simulink model "FluidAndThermodynamics_simulink"  (R2022a)
settings: Solver=VariableStepAuto  StartTime=0.0  StopTime=10.0  RelTol=1e-3
settings Model: Creator=Anupp  LastModifiedBy=Anupp

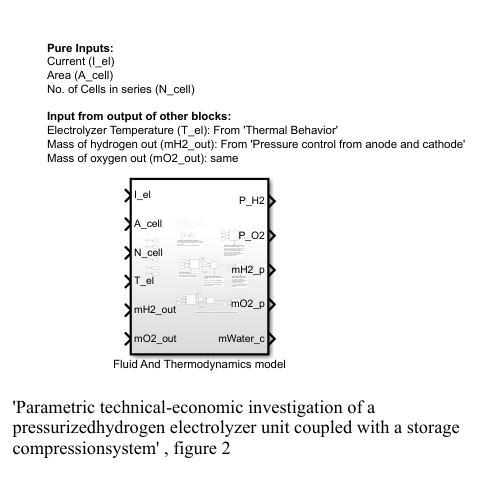
[thumbnail: Simulink's stored preview of the top-level diagram]
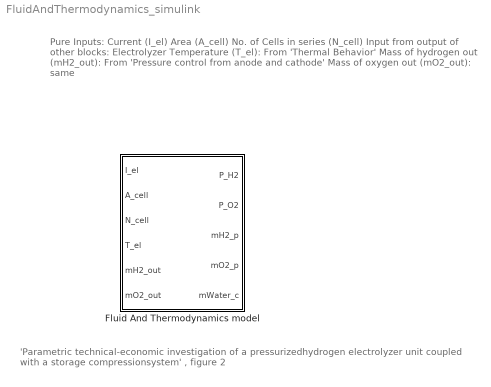
== system FluidAndThermodynamics_simulink ==
  note: Pure Inputs:
      | Current (I_el)
      | Area (A_cell)
      | No. of Cells in series (N_cell)
      |
      | Input from output of other blocks:
      | Electrolyzer Temperature (T_el): From 'Thermal Behavior'
      | Mass of hydrogen out (mH2_out): From 'Pressure control from anode and cathode'
      | Mass of oxygen out (mO2_out): same
  note: 'Parametric technical-economic investigation of a pressurizedhydrogen electrolyzer unit coupled with a storage compressionsystem' , figure 2
  Fluid And Thermodynamics model : Subsystem  TreatAsAtomicUnit=on

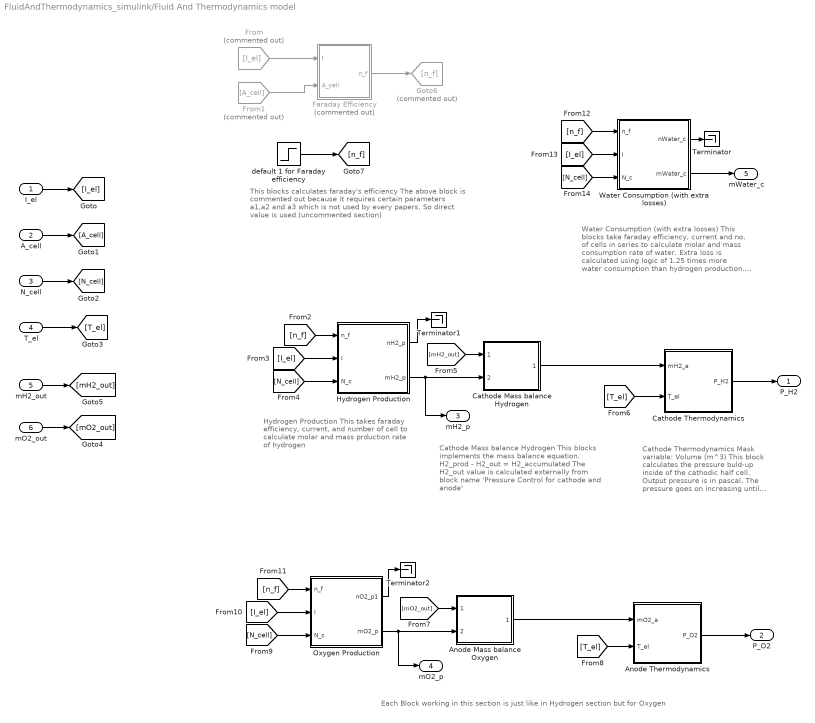
== system FluidAndThermodynamics_simulink/Fluid And Thermodynamics model ==
  note: Water Consumption (with extra losses)
      | This blocks take faraday efficiency, current and no. of cells in series to calculate molar and mass consumption rate of water.
      | Extra loss is calculated using logic of 1.25 times more water consumption than hydrogen production. Ideally, same moles of hydrgen production and water consumption takes place.
  note: This blocks calculates faraday's efficiency
      | The above block is commented out because it requires certain parameters a1,a2 and a3 which is not used by every papers.
      | So direct value is used (uncommented section)
  note: Each Block working in this section is just like in Hydrogen section but for Oxygen
  note: Cathode Thermodynamics
      | Mask variable: Volume (m^3)
      | This block calculates the pressure buld-up inside of the cathodic half cell. Output pressure is in pascal.
      | The pressure goes on increasing until the nominal pressure is reached.
  note: Cathode Mass balance Hydrogen
      | This blocks implements the mass balance equation.
      | H2_prod - H2_out = H2_accumulated
      |
      | The H2_out value is calculated externally from block name 'Pressure Control for cathode and anode'
  note: Hydrogen Production
      | This takes faraday efficiency, current, and number of cell to calculate molar and mass prduction rate of hydrogen
  I_el : Inport
  A_cell : Inport  Port=2
  N_cell : Inport  Port=3
  T_el : Inport  Port=4
  mH2_out : Inport  Port=5
  mO2_out : Inport  Port=6
  Anode Mass balance Oxygen : Subsystem
  Anode Thermodynamics : Subsystem  mask{V=0}
      mask prompts: V "Anode Volume"
  Cathode Mass balance Hydrogen : Subsystem
  Cathode Thermodynamics : Subsystem  mask{V=0}
      mask prompts: V "Cathode Volume"
  Faraday Efficiency : Subsystem  Commented=on  mask{a1=0, a2=0, a3=0}
      mask DialogControl DescTextVar Prompt: Define Faraday's efficiency parameters for alkaline electrolyser
  From : From  Commented=on  GotoTag=I_el
  From1 : From  Commented=on  GotoTag=A_cell
  Goto6 : Goto  Commented=on  GotoTag=n_f
  Hydrogen Production : Subsystem
  Oxygen Production : Subsystem
  Terminator : Terminator
  Terminator1 : Terminator
  Terminator2 : Terminator
  Water Consumption (with extra losses) : Subsystem
  default 1 for Faraday efficiency : Step  Time=0  SampleTime=0
  P_H2 : Outport
  P_O2 : Outport  Port=2
  mH2_p : Outport  Port=3
  mO2_p : Outport  Port=4
  mWater_c : Outport  Port=5
  wires:
  From1/1 -> Faraday Efficiency/2(A_cell)
  From/1 -> Faraday Efficiency/1(I)
  Cathode Mass balance Hydrogen/1(mH2_a) -> Cathode Thermodynamics/1(mH2_a)
  [n_f] -> Hydrogen Production/1(n_f)
  T_el/1 -> [T_el]
  [I_el] -> Water Consumption (with extra losses)/2(I)
  Hydrogen Production/2(mH2_p) -> mH2_p/1, Cathode Mass balance Hydrogen/2(mH2_p)
  N_cell/1 -> [N_cell]
  I_el/1 -> [I_el]
  [n_f] -> Oxygen Production/1(n_f)
  mO2_out/1 -> [mO2_out]
  Water Consumption (with extra losses)/2(mWater_c) -> mWater_c/1
  A_cell/1 -> [A_cell]
  mH2_out/1 -> [mH2_out]
  [I_el] -> Oxygen Production/2(I)
  [N_cell] -> Oxygen Production/3(N_c)
  [mH2_out] -> Cathode Mass balance Hydrogen/1(mH2_out)
  [N_cell] -> Hydrogen Production/3(N_c)
  Oxygen Production/2(mO2_p) -> mO2_p/1, Anode Mass balance Oxygen/2(mO2_p)
  [I_el] -> Hydrogen Production/2(I)
  Faraday Efficiency/1(n_f) -> Goto6/1
  [T_el] -> Cathode Thermodynamics/2(T_el)
  [N_cell] -> Water Consumption (with extra losses)/3(N_c)
  [n_f] -> Water Consumption (with extra losses)/1(n_f)
  [T_el] -> Anode Thermodynamics/2(T_el)
  Anode Mass balance Oxygen/1(mO2_a) -> Anode Thermodynamics/1(mO2_a)
  [mO2_out] -> Anode Mass balance Oxygen/1(mO2_out)
  Cathode Thermodynamics/1(P_H2) -> P_H2/1
  Anode Thermodynamics/1(P_O2) -> P_O2/1
  Water Consumption (with extra losses)/1(nWater_c) -> Terminator/1
  Hydrogen Production/1(nH2_p) -> Terminator1/1
  Oxygen Production/1(nO2_p1) -> Terminator2/1
  default 1 for Faraday efficiency/1 -> [n_f]

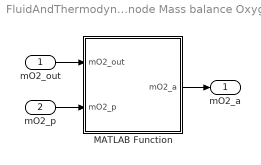
== system FluidAndThermodynamics_simulink/Fluid And Thermodynamics model/Anode Mass balance Oxygen ==
  mO2_out : Inport
  mO2_p : Inport  Port=2
  MATLAB Function : MATLAB Function  TreatAsAtomicUnit=on
  mO2_a : Outport
  wires:
  MATLAB Function/1(mO2_a) -> mO2_a/1
  mO2_p/1 -> MATLAB Function/2(mO2_p)
  mO2_out/1 -> MATLAB Function/1(mO2_out)

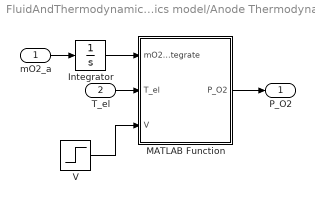
== system FluidAndThermodynamics_simulink/Fluid And Thermodynamics model/Anode Thermodynamics ==
  mO2_a : Inport
  T_el : Inport  Port=2
  Integrator : Integrator
  MATLAB Function : MATLAB Function  TreatAsAtomicUnit=on
  V : Step  Time=0  After=V  SampleTime=0
  P_O2 : Outport
  wires:
  T_el/1 -> MATLAB Function/2(T_el)
  mO2_a/1 -> Integrator/1
  Integrator/1 -> MATLAB Function/1(mO2_a_integrate)
  MATLAB Function/1(P_O2) -> P_O2/1
  V/1 -> MATLAB Function/3(V)

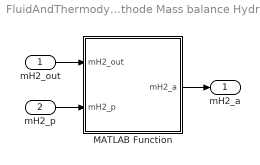
== system FluidAndThermodynamics_simulink/Fluid And Thermodynamics model/Cathode Mass balance Hydrogen ==
  mH2_out : Inport
  mH2_p : Inport  Port=2
  MATLAB Function : MATLAB Function  TreatAsAtomicUnit=on
  mH2_a : Outport
  wires:
  MATLAB Function/1(mH2_a) -> mH2_a/1
  mH2_p/1 -> MATLAB Function/2(mH2_p)
  mH2_out/1 -> MATLAB Function/1(mH2_out)

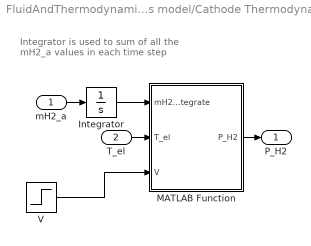
== system FluidAndThermodynamics_simulink/Fluid And Thermodynamics model/Cathode Thermodynamics ==
  note: Integrator is used to sum of all the mH2_a values in each time step
  mH2_a : Inport
  T_el : Inport  Port=2
  Integrator : Integrator
  MATLAB Function : MATLAB Function  TreatAsAtomicUnit=on
  V : Step  Time=0  After=V  SampleTime=0
  P_H2 : Outport
  wires:
  Integrator/1 -> MATLAB Function/1(mH2_a_integrate)
  MATLAB Function/1(P_H2) -> P_H2/1
  mH2_a/1 -> Integrator/1
  T_el/1 -> MATLAB Function/2(T_el)
  V/1 -> MATLAB Function/3(V)

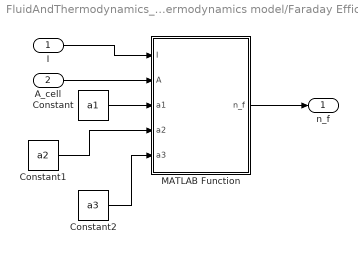
== system FluidAndThermodynamics_simulink/Fluid And Thermodynamics model/Faraday Efficiency ==
  I : Inport
  A_cell : Inport  Port=2
  Constant : Constant  Value=a1
  Constant1 : Constant  Value=a2
  Constant2 : Constant  Value=a3
  MATLAB Function : MATLAB Function  TreatAsAtomicUnit=on
  n_f : Outport
  wires:
  MATLAB Function/1(n_f) -> n_f/1
  Constant2/1 -> MATLAB Function/5(a3)
  Constant1/1 -> MATLAB Function/4(a2)
  A_cell/1 -> MATLAB Function/2(A)
  I/1 -> MATLAB Function/1(I)
  Constant/1 -> MATLAB Function/3(a1)

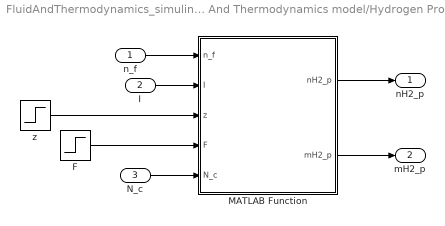
== system FluidAndThermodynamics_simulink/Fluid And Thermodynamics model/Hydrogen Production ==
  n_f : Inport
  I : Inport  Port=2
  N_c : Inport  Port=3
  F : Step  Time=0  After=96485  SampleTime=0
  MATLAB Function : MATLAB Function  TreatAsAtomicUnit=on
  z : Step  Time=0  After=2  SampleTime=0
  nH2_p : Outport
  mH2_p : Outport  Port=2
  wires:
  n_f/1 -> MATLAB Function/1(n_f)
  I/1 -> MATLAB Function/2(I)
  MATLAB Function/2(mH2_p) -> mH2_p/1
  N_c/1 -> MATLAB Function/5(N_c)
  F/1 -> MATLAB Function/4(F)
  z/1 -> MATLAB Function/3(z)
  MATLAB Function/1(nH2_p) -> nH2_p/1

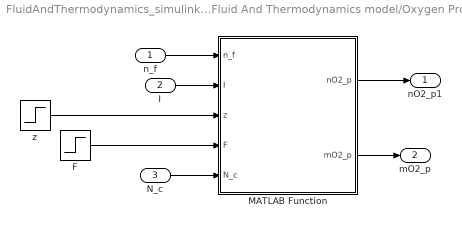
== system FluidAndThermodynamics_simulink/Fluid And Thermodynamics model/Oxygen Production ==
  n_f : Inport
  I : Inport  Port=2
  N_c : Inport  Port=3
  F : Step  Time=0  After=96485  SampleTime=0
  MATLAB Function : MATLAB Function  TreatAsAtomicUnit=on
  z : Step  Time=0  After=2  SampleTime=0
  nO2_p1 : Outport
  mO2_p : Outport  Port=2
  wires:
  n_f/1 -> MATLAB Function/1(n_f)
  I/1 -> MATLAB Function/2(I)
  MATLAB Function/2(mO2_p) -> mO2_p/1
  N_c/1 -> MATLAB Function/5(N_c)
  MATLAB Function/1(nO2_p) -> nO2_p1/1
  F/1 -> MATLAB Function/4(F)
  z/1 -> MATLAB Function/3(z)

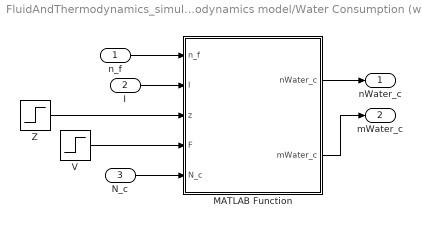
== system FluidAndThermodynamics_simulink/Fluid And Thermodynamics model/Water Consumption (with extra losses) ==
  n_f : Inport
  I : Inport  Port=2
  N_c : Inport  Port=3
  MATLAB Function : MATLAB Function  TreatAsAtomicUnit=on
  V : Step  Time=0  After=96485  SampleTime=0
  Z : Step  Time=0  After=2  SampleTime=0
  nWater_c : Outport
  mWater_c : Outport  Port=2
  wires:
  n_f/1 -> MATLAB Function/1(n_f)
  I/1 -> MATLAB Function/2(I)
  MATLAB Function/2(mWater_c) -> mWater_c/1
  N_c/1 -> MATLAB Function/5(N_c)
  MATLAB Function/1(nWater_c) -> nWater_c/1
  Z/1 -> MATLAB Function/3(z)
  V/1 -> MATLAB Function/4(F)

== matlab function FluidAndThermodynamics_simulink/Fluid And Thermodynamics model/Hydrogen Production/MATLAB Function ==
  data: nH2_p output; n_f input; mH2_p output; I input; z input; F input; N_c input
%% Inputs:
% Faraday's Efficiency (n_f)
% Current (I): A
% Number of elctrons that take part in electrolysis (z): 2 for this
% Faraday's constant (F): 96485 C mol^-1
% number of cells in series (N_c)

%% Outputs:
% moles of hydrogen per second (nH2): mol/s
% mass of hydrogen per second (mH2): kg/s



function [nH2_p,mH2_p] = fcn(n_f,I,z,F,N_c)

nH2_p = n_f * I * N_c / (z * F);
mH2_p = 2.016 * 1e-3 * nH2_p; 

end

== matlab function FluidAndThermodynamics_simulink/Fluid And Thermodynamics model/Faraday Efficiency/MATLAB Function ==
  data: I input; n_f output; A input; a1 input; a2 input; a3 input
%% Inputs:
% Current (I): Ampere
% Area (A): m^2
% a1,a2,a3 parameters

%% Output:
% Faraday's Efficiency (n_f)

%% Main Function

function n_f = fcn(I,A,a1,a2,a3)

n_f = a1 .* exp(a2/(I/A) + a3/(I/A)^2);

end

== matlab function FluidAndThermodynamics_simulink/Fluid And Thermodynamics model/Oxygen Production/MATLAB Function ==
  data: nO2_p output; n_f input; mO2_p output; I input; z input; F input; N_c input
function [nO2_p,mO2_p] = fcn(n_f,I,z,F,N_c)

nO2_p = 0.5 * n_f * I * N_c / (z * F);

mO2_p = 32 * 1e-3 * nO2_p;

end

== matlab function FluidAndThermodynamics_simulink/Fluid And Thermodynamics model/Water Consumption (with extra losses)/MATLAB Function ==
  data: nWater_c output; n_f input; mWater_c output; I input; z input; F input; N_c input
%% Inputs:
% Faraday's Efficiency (n_f)
% Current(I): Ampere
% z:2
% Faraday's constant (F): 96485 C mol^-1
% No. of cells in series (N_c)

%% Outputs:
% molar consumption of water (nWater_c): mol/s
% Mass consumption of water (mWater_c): kg/s

%% Main Function (1.25 is used for extra 0.25 losses due to leakages)
function [nWater_c,mWater_c] = fcn(n_f,I,z,F,N_c)

nWater_c = 1.25 * n_f * I * N_c / (z * F);

mWater_c = 18.015 * 1e-3 * nWater_c;

end

== matlab function FluidAndThermodynamics_simulink/Fluid And Thermodynamics model/Cathode Mass balance Hydrogen/MATLAB Function ==
  data: mH2_out input; mH2_a output; mH2_p input
%% Inputs:
% Hydrogen out of the electrolyzer (mH2_out): kg/s
% Hydrogen produced                (mH2_p)  : kg/s

%% Output:
% Hydrogen accumulated at the electrolyzer (mH2_a): kg/s

%% Main function

function mH2_a  = fcn(mH2_out,mH2_p)

mH2_a = mH2_p - mH2_out;

end

== matlab function FluidAndThermodynamics_simulink/Fluid And Thermodynamics model/Cathode Thermodynamics/MATLAB Function ==
  data: mH2_a_integrate input; P_H2 output; T_el input; V input
%% Inputs:
% Integrated value of mH2_a (integration function adds up mH2 in each time
% step: Kg
% Electrolyzer Temeperature (T_el): Kelvin
% Volume (V): m^3

%% Output:
% Pressure of Hydrogen inside electrolyzer (P_H2): N m^-3 or Pascal

%% Main function

function P_H2 = fcn(mH2_a_integrate,T_el, V)

P_H2 =  (8.3143 * T_el)/(V*2.016*(1e-3)) * mH2_a_integrate;

end

== matlab function FluidAndThermodynamics_simulink/Fluid And Thermodynamics model/Anode Mass balance Oxygen/MATLAB Function ==
  data: mO2_out input; mO2_a output; mO2_p input
function mO2_a  = fcn(mO2_out,mO2_p)

mO2_a = mO2_p - mO2_out;

end

== matlab function FluidAndThermodynamics_simulink/Fluid And Thermodynamics model/Anode Thermodynamics/MATLAB Function ==
  data: mO2_a_integrate input; P_O2 output; T_el input; V input
function P_O2 = fcn(mO2_a_integrate,T_el, V)

P_O2 =  (8.3143 * T_el)/(V*32*(1e-3)) * mO2_a_integrate;

end
